simulink model "VIPL557LTStEnCtrl"  (R2024b)
settings: Solver=FixedStepDiscrete  StartTime=0.0  StopTime=10.0  RelTol=1e-3
undefined symbols (not defined in the file or in its folder): data, KeSMSw4SSecRwLtStLgrstUpwdDnwdOpenPos1_Val, SecRwLtStBkReclnEn_Clear, SecRwLtStBkReclnEn_Set, SecRwLtStFwdBkwdEn_Clear, SecRwLtStFwdBkwdEn_Set, SecRwLtStLgrstInwdOtwdEn_Clear, SecRwLtStLgrstInwdOtwdEn_Set, SecRwLtStLgrstUpwdDnwdEn_Clear, SecRwLtStLgrstUpwdDnwdEn_Set, ThdRwLtStBkReclnEn_Clear, ThdRwLtStBkReclnEn_Set, ThdRwLtStFwdBkwdEn_Clear, ThdRwLtStFwdBkwdEn_Set
libraries: simulink x1
settings Model: ModifiedHistory=2024.6.28 V3.0.0 座椅模式流程图V1.9  Creator=sn2xws  LastModifiedBy=sn55gm
settings SolverCC: AlgebraicLoopSolver=TrustRegion
settings DataIOCC: SaveFormat=StructureWithTime  ReturnWorkspaceOutputs=off
settings OptimizationCC: DefaultParameterBehavior=Inlined  EnhancedBackFolding=on  PassReuseOutputArgsAs=Individual arguments  ZeroExternalMemoryAtStartup=off  ZeroInternalMemoryAtStartup=off  OptimizeBlockOrder=speed  DifferentSizesBufferReuse=on  OptimizationCustomize=off  EfficientTunableParamExpr=on
settings DebuggingCC: ParameterTunabilityLossMsg=error  UnconnectedInputMsg=warning  UnconnectedOutputMsg=warning  UnconnectedLineMsg=warning  ArithmeticOperatorsInVariantConditions=warning
settings ModelReferenceCC: EnableRefExpFcnMdlSchedulingChecks=on
settings SFSimCC: MATLABDynamicMemAlloc=off  CustomCodeUndefinedFunction=UseInterfaceOnly
settings RTWCC: Description=AUTOSAR  SystemTargetFile=autosar.tlc  GenCodeOnly=on  TemplateMakefile=ert_default_tmf  GenerateReport=on  IncludeHyperlinkInReport=on  LaunchReport=on  DataTypeReplacement=CDataTypesFixedWidth  GenerateTraceInfo=on  GenerateTraceReport=on  GenerateTraceReportSl=on  GenerateTraceReportSf=on  GenerateTraceReportEml=on  GPUComputeCapability=3.5
settings CodeAppCC: ForceParamTrailComments=on  IgnoreCustomStorageClasses=off  OperatorAnnotations=on  SimulinkDataObjDesc=on  SFDataObjDesc=on  InsertBlockDesc=on
settings STFCustomTargetCC: TargetLangStandard=C99 (ISO)  MultiwordLength=256  ParMdlRefBuildCompliant=on  CompOptLevelCompliant=on  IncludeMdlTerminateFcn=off  CombineOutputUpdateFcns=on  SuppressErrorStatus=on  ERTCustomFileBanners=on  SupportNonFinite=off  SupportComplex=off  SupportContinuousTime=off  SupportNonInlinedSFcns=off  RemoveResetFunc=on  MATLABClassNameForMDSCustomization=Simulink.SoftwareTarget.ERTCustomization  AutosarCompliant=on  UseToolchainInfoCompliant=on  LookupTableObjectStructAxisOrder=2,1,3,4,...  LUTObjectStructOrderEvenSpacing=Size,Table,Breakpoints  SystemTargetFile=autosar.tlc
settings ERTTargetCC: TargetLangStandard=C99 (ISO)  ConcurrentExecutionCompliant=off  IncludeMdlTerminateFcn=off  SuppressErrorStatus=on  SupportNonFinite=off  SupportComplex=off  ModelStepFunctionPrototypeControlCompliant=off  CPPClassGenCompliant=off  AutosarCompliant=on  LookupTableObjectStructAxisOrder=2,1,3,4,...  LUTObjectStructOrderEvenSpacing=Size,Table,Breakpoints  ERTCustomFileTemplate=example_file_process.tlc  ERTFilePackagingFormat=Compact  BooleanTrueId=TRUE  BooleanFalseId=FALSE  DynamicArrayContainerType=coder::array

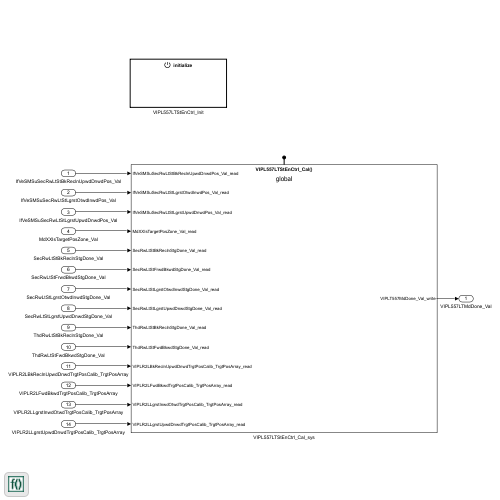
[thumbnail: Simulink's stored preview of the top-level diagram]
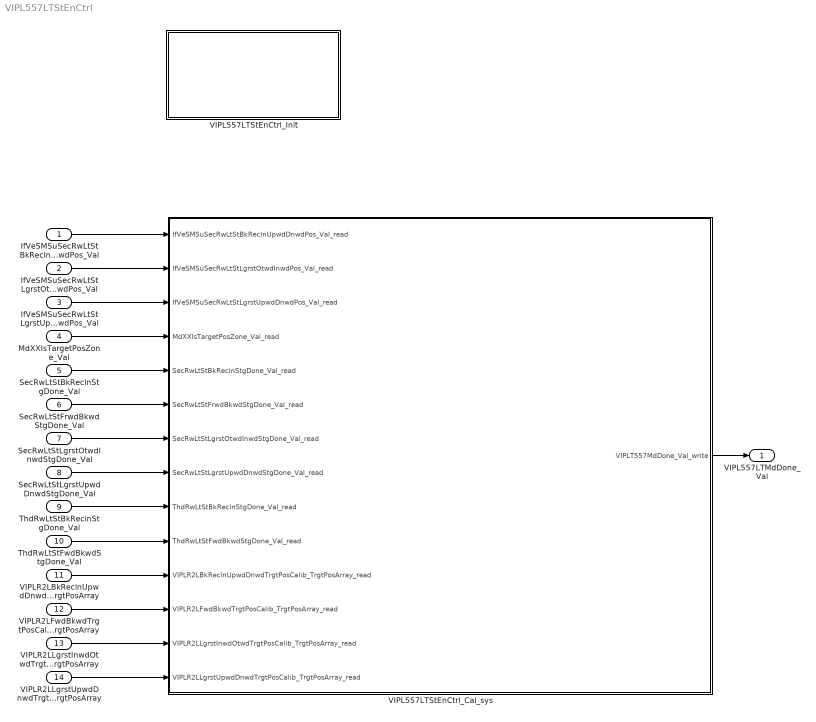
== system VIPL557LTStEnCtrl ==
  IfVeSMSuSecRwLtStBkReclnUpwdDnwdPos_Val : Inport  OutDataTypeStr=uint16  PortDimensions=1
  IfVeSMSuSecRwLtStLgrstOtwdInwdPos_Val : Inport  Port=2  OutDataTypeStr=uint16  PortDimensions=1
  IfVeSMSuSecRwLtStLgrstUpwdDnwdPos_Val : Inport  Port=3  OutDataTypeStr=uint16  PortDimensions=1
  MdXXIsTargetPosZone_Val : Inport  Port=4  OutDataTypeStr=uint32  PortDimensions=1
  SecRwLtStBkReclnStgDone_Val : Inport  Port=5  OutDataTypeStr=boolean  PortDimensions=1
  SecRwLtStFrwdBkwdStgDone_Val : Inport  Port=6  OutDataTypeStr=boolean  PortDimensions=1
  SecRwLtStLgrstOtwdInwdStgDone_Val : Inport  Port=7  OutDataTypeStr=boolean  PortDimensions=1
  SecRwLtStLgrstUpwdDnwdStgDone_Val : Inport  Port=8  OutDataTypeStr=boolean  PortDimensions=1
  ThdRwLtStBkReclnStgDone_Val : Inport  Port=9  OutDataTypeStr=boolean  PortDimensions=1
  ThdRwLtStFwdBkwdStgDone_Val : Inport  Port=10  OutDataTypeStr=boolean  PortDimensions=1
  VIPLR2LBkReclnUpwdDnwdTrgtPosCalib_TrgtPosArray : Inport  Description=|  Port=11  OutDataTypeStr=uint16  PortDimensions=3
      | 0:Pos
      | 1:Max
      | 2:Min
  VIPLR2LFwdBkwdTrgtPosCalib_TrgtPosArray : Inport  Description=|  Port=12  OutDataTypeStr=uint16  PortDimensions=3
      | 0:Pos
      | 1:Max
      | 2:Min
  VIPLR2LLgrstInwdOtwdTrgtPosCalib_TrgtPosArray : Inport  Description=|  Port=13  OutDataTypeStr=uint16  PortDimensions=3
      | 0:Pos
      | 1:Max
      | 2:Min
  VIPLR2LLgrstUpwdDnwdTrgtPosCalib_TrgtPosArray : Inport  Description=|  Port=14  OutDataTypeStr=uint16  PortDimensions=3
      | 0:Pos
      | 1:Max
      | 2:Min
  VIPL557LTStEnCtrl_Cal_sys : Subsystem
  VIPL557LTStEnCtrl_Init : Subsystem
  VIPL557LTMdDone_Val : Outport  OutDataTypeStr=uint8  PortDimensions=1  VectorParamsAs1DForOutWhenUnconnected=off
  wires:
  IfVeSMSuSecRwLtStBkReclnUpwdDnwdPos_Val/1 -> VIPL557LTStEnCtrl_Cal_sys/1(IfVeSMSuSecRwLtStBkReclnUpwdDnwdPos_Val_read)
  IfVeSMSuSecRwLtStLgrstOtwdInwdPos_Val/1 -> VIPL557LTStEnCtrl_Cal_sys/2(IfVeSMSuSecRwLtStLgrstOtwdInwdPos_Val_read)
  IfVeSMSuSecRwLtStLgrstUpwdDnwdPos_Val/1 -> VIPL557LTStEnCtrl_Cal_sys/3(IfVeSMSuSecRwLtStLgrstUpwdDnwdPos_Val_read)
  MdXXIsTargetPosZone_Val/1 -> VIPL557LTStEnCtrl_Cal_sys/4(MdXXIsTargetPosZone_Val_read)
  SecRwLtStBkReclnStgDone_Val/1 -> VIPL557LTStEnCtrl_Cal_sys/5(SecRwLtStBkReclnStgDone_Val_read)
  SecRwLtStFrwdBkwdStgDone_Val/1 -> VIPL557LTStEnCtrl_Cal_sys/6(SecRwLtStFrwdBkwdStgDone_Val_read)
  SecRwLtStLgrstOtwdInwdStgDone_Val/1 -> VIPL557LTStEnCtrl_Cal_sys/7(SecRwLtStLgrstOtwdInwdStgDone_Val_read)
  SecRwLtStLgrstUpwdDnwdStgDone_Val/1 -> VIPL557LTStEnCtrl_Cal_sys/8(SecRwLtStLgrstUpwdDnwdStgDone_Val_read)
  ThdRwLtStBkReclnStgDone_Val/1 -> VIPL557LTStEnCtrl_Cal_sys/9(ThdRwLtStBkReclnStgDone_Val_read)
  ThdRwLtStFwdBkwdStgDone_Val/1 -> VIPL557LTStEnCtrl_Cal_sys/10(ThdRwLtStFwdBkwdStgDone_Val_read)
  VIPLR2LBkReclnUpwdDnwdTrgtPosCalib_TrgtPosArray/1 -> VIPL557LTStEnCtrl_Cal_sys/11(VIPLR2LBkReclnUpwdDnwdTrgtPosCalib_TrgtPosArray_read)
  VIPLR2LFwdBkwdTrgtPosCalib_TrgtPosArray/1 -> VIPL557LTStEnCtrl_Cal_sys/12(VIPLR2LFwdBkwdTrgtPosCalib_TrgtPosArray_read)
  VIPLR2LLgrstInwdOtwdTrgtPosCalib_TrgtPosArray/1 -> VIPL557LTStEnCtrl_Cal_sys/13(VIPLR2LLgrstInwdOtwdTrgtPosCalib_TrgtPosArray_read)
  VIPLR2LLgrstUpwdDnwdTrgtPosCalib_TrgtPosArray/1 -> VIPL557LTStEnCtrl_Cal_sys/14(VIPLR2LLgrstUpwdDnwdTrgtPosCalib_TrgtPosArray_read)
  VIPL557LTStEnCtrl_Cal_sys/1(VIPLT557MdDone_Val_write) -> VIPL557LTMdDone_Val/1

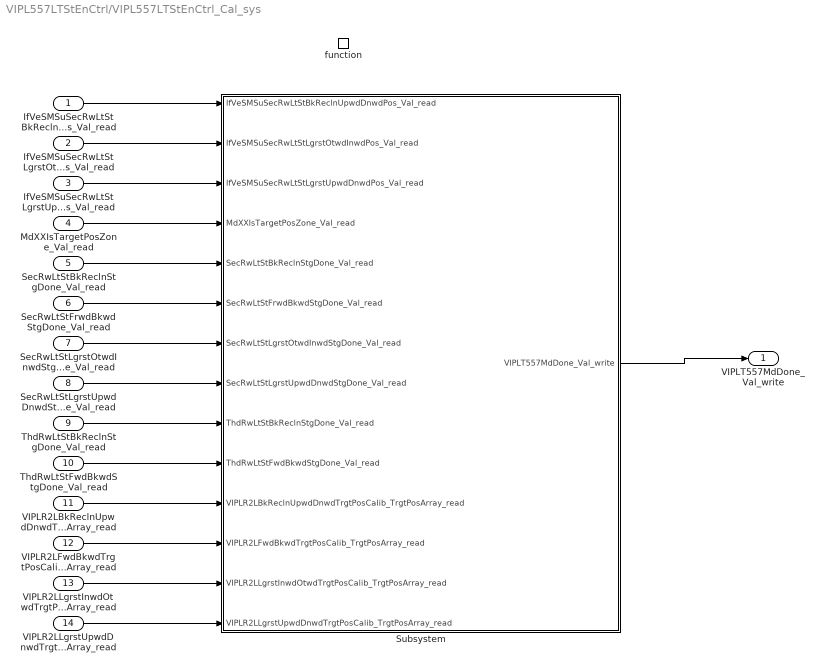
== system VIPL557LTStEnCtrl/VIPL557LTStEnCtrl_Cal_sys ==
  IfVeSMSuSecRwLtStBkReclnUpwdDnwdPos_Val_read : Inport
  IfVeSMSuSecRwLtStLgrstOtwdInwdPos_Val_read : Inport  Port=2
  IfVeSMSuSecRwLtStLgrstUpwdDnwdPos_Val_read : Inport  Port=3
  MdXXIsTargetPosZone_Val_read : Inport  Port=4
  SecRwLtStBkReclnStgDone_Val_read : Inport  Port=5
  SecRwLtStFrwdBkwdStgDone_Val_read : Inport  Port=6
  SecRwLtStLgrstOtwdInwdStgDone_Val_read : Inport  Port=7
  SecRwLtStLgrstUpwdDnwdStgDone_Val_read : Inport  Port=8
  ThdRwLtStBkReclnStgDone_Val_read : Inport  Port=9
  ThdRwLtStFwdBkwdStgDone_Val_read : Inport  Port=10
  VIPLR2LBkReclnUpwdDnwdTrgtPosCalib_TrgtPosArray_read : Inport  Port=11
  VIPLR2LFwdBkwdTrgtPosCalib_TrgtPosArray_read : Inport  Port=12
  VIPLR2LLgrstInwdOtwdTrgtPosCalib_TrgtPosArray_read : Inport  Port=13
  VIPLR2LLgrstUpwdDnwdTrgtPosCalib_TrgtPosArray_read : Inport  Port=14
  function : TriggerPort  TriggerType=function-call  IsSimulinkFunction=on  FunctionName=VIPL557LTStEnCtrl_Cal  VariantControl=(inherit)
  Subsystem : Subsystem
  VIPLT557MdDone_Val_write : Outport  VectorParamsAs1DForOutWhenUnconnected=off
      settings: EnsureOutportIsVirtual=on
  wires:
  IfVeSMSuSecRwLtStBkReclnUpwdDnwdPos_Val_read/1 -> Subsystem/1(IfVeSMSuSecRwLtStBkReclnUpwdDnwdPos_Val_read)
  IfVeSMSuSecRwLtStLgrstOtwdInwdPos_Val_read/1 -> Subsystem/2(IfVeSMSuSecRwLtStLgrstOtwdInwdPos_Val_read)
  IfVeSMSuSecRwLtStLgrstUpwdDnwdPos_Val_read/1 -> Subsystem/3(IfVeSMSuSecRwLtStLgrstUpwdDnwdPos_Val_read)
  MdXXIsTargetPosZone_Val_read/1 -> Subsystem/4(MdXXIsTargetPosZone_Val_read)
  SecRwLtStBkReclnStgDone_Val_read/1 -> Subsystem/5(SecRwLtStBkReclnStgDone_Val_read)
  SecRwLtStFrwdBkwdStgDone_Val_read/1 -> Subsystem/6(SecRwLtStFrwdBkwdStgDone_Val_read)
  SecRwLtStLgrstOtwdInwdStgDone_Val_read/1 -> Subsystem/7(SecRwLtStLgrstOtwdInwdStgDone_Val_read)
  SecRwLtStLgrstUpwdDnwdStgDone_Val_read/1 -> Subsystem/8(SecRwLtStLgrstUpwdDnwdStgDone_Val_read)
  ThdRwLtStBkReclnStgDone_Val_read/1 -> Subsystem/9(ThdRwLtStBkReclnStgDone_Val_read)
  ThdRwLtStFwdBkwdStgDone_Val_read/1 -> Subsystem/10(ThdRwLtStFwdBkwdStgDone_Val_read)
  VIPLR2LBkReclnUpwdDnwdTrgtPosCalib_TrgtPosArray_read/1 -> Subsystem/11(VIPLR2LBkReclnUpwdDnwdTrgtPosCalib_TrgtPosArray_read)
  VIPLR2LFwdBkwdTrgtPosCalib_TrgtPosArray_read/1 -> Subsystem/12(VIPLR2LFwdBkwdTrgtPosCalib_TrgtPosArray_read)
  VIPLR2LLgrstInwdOtwdTrgtPosCalib_TrgtPosArray_read/1 -> Subsystem/13(VIPLR2LLgrstInwdOtwdTrgtPosCalib_TrgtPosArray_read)
  VIPLR2LLgrstUpwdDnwdTrgtPosCalib_TrgtPosArray_read/1 -> Subsystem/14(VIPLR2LLgrstUpwdDnwdTrgtPosCalib_TrgtPosArray_read)
  Subsystem/1(VIPLT557MdDone_Val_write) -> VIPLT557MdDone_Val_write/1

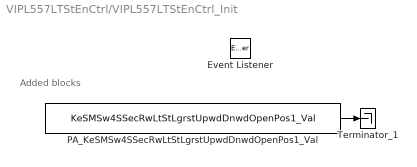
== system VIPL557LTStEnCtrl/VIPL557LTStEnCtrl_Init ==
  note: Added blocks
  Event Listener : EventListener  EventName=reset
  PA_KeSMSw4SSecRwLtStLgrstUpwdDnwdOpenPos1_Val : Constant  Value=KeSMSw4SSecRwLtStLgrstUpwdDnwdOpenPos1_Val
  Terminator_1 : Terminator
  wires:
  PA_KeSMSw4SSecRwLtStLgrstUpwdDnwdOpenPos1_Val/1 -> Terminator_1/1

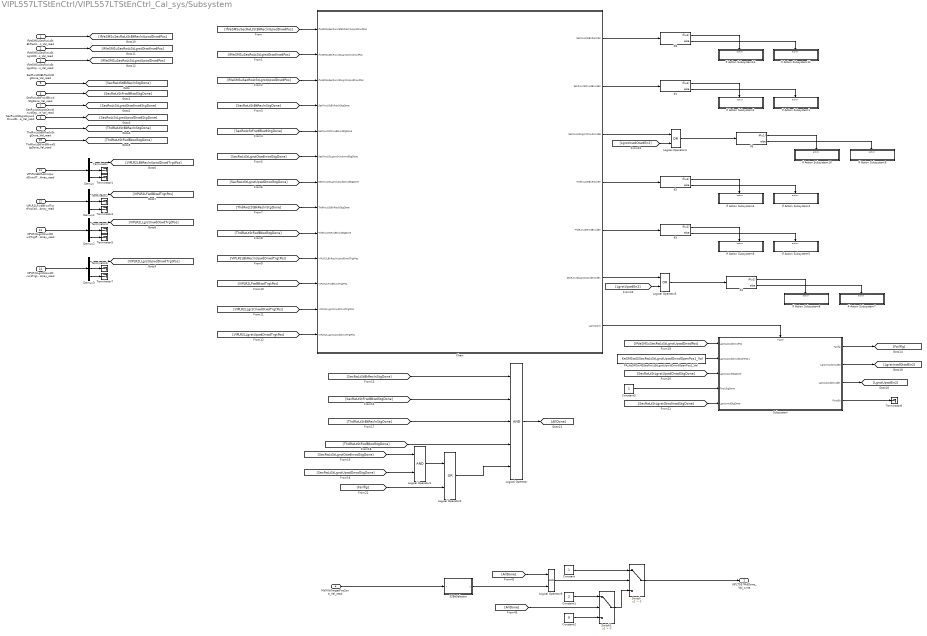
== system VIPL557LTStEnCtrl/VIPL557LTStEnCtrl_Cal_sys/Subsystem ==
  IfVeSMSuSecRwLtStBkReclnUpwdDnwdPos_Val_read : Inport
  IfVeSMSuSecRwLtStLgrstOtwdInwdPos_Val_read : Inport  Port=2
  IfVeSMSuSecRwLtStLgrstUpwdDnwdPos_Val_read : Inport  Port=3
  MdXXIsTargetPosZone_Val_read : Inport  Port=4
  SecRwLtStBkReclnStgDone_Val_read : Inport  Port=5
  SecRwLtStFrwdBkwdStgDone_Val_read : Inport  Port=6
  SecRwLtStLgrstOtwdInwdStgDone_Val_read : Inport  Port=7
  SecRwLtStLgrstUpwdDnwdStgDone_Val_read : Inport  Port=8
  ThdRwLtStBkReclnStgDone_Val_read : Inport  Port=9
  ThdRwLtStFwdBkwdStgDone_Val_read : Inport  Port=10
  VIPLR2LBkReclnUpwdDnwdTrgtPosCalib_TrgtPosArray_read : Inport  Port=11
  VIPLR2LFwdBkwdTrgtPosCalib_TrgtPosArray_read : Inport  Port=12
  VIPLR2LLgrstInwdOtwdTrgtPosCalib_TrgtPosArray_read : Inport  Port=13
  VIPLR2LLgrstUpwdDnwdTrgtPosCalib_TrgtPosArray_read : Inport  Port=14
  32BitSelector : Subsystem  mask(32 Bit Selector){BitNum=9}
      mask prompts: BitNum "Select Bit Number"
      mask help: Allows selection of a particular bit (0-31) out of a packed word up to 32 bits long. Output will be true if the bit number selected via the mask parameter is equal to one.
      mask TypeOptions BitNum: 0 | 1 | 2 | 3 | 4 | 5 | 6 | 7 | 8 | 9 | 10 | 11 | 12 | 13 | 14 | 15 | 16 | 17 | 18 | 19 | 20 | 21 | 22 | 23 | 24 | 25 | 26 | 27 | 28 | 29 | 30 | 31
      mask Display:
      | text(0.5, 0.8,'BIT','horizontalAlignment','center')
      | text(0.5, 0.5,'SELECTOR','horizontalAlignment','center')
      | text(0.5, 0.2,['-- Bit ',char(get_param(gcb,'BitNum')),' --'],'horizontalAlignment','center')
  Chart : Stateflow chart  TreatAsAtomicUnit=on
  Constant : Constant  OutDataTypeStr=uint8
  Constant1 : Constant  Value=2  OutDataTypeStr=uint8
  Constant2 : Constant  Value=0  OutDataTypeStr=uint8
  Constant3 : Constant  OutDataTypeStr=boolean
  Demux{,1..3} (4 alike) : Demux  Outputs=3
  If Action Subsystem1 : Subsystem  TreatAsAtomicUnit=on
  If Action Subsystem10 : Subsystem  TreatAsAtomicUnit=on
  If Action Subsystem11 : Subsystem  TreatAsAtomicUnit=on
  If Action Subsystem14 : Subsystem  TreatAsAtomicUnit=on
  If Action Subsystem2 : Subsystem  TreatAsAtomicUnit=on
  If Action Subsystem3 : Subsystem  TreatAsAtomicUnit=on
  If Action Subsystem4 : Subsystem  TreatAsAtomicUnit=on
  If Action Subsystem5 : Subsystem  TreatAsAtomicUnit=on
  If Action Subsystem6 : Subsystem  TreatAsAtomicUnit=on
  If Action Subsystem7 : Subsystem  TreatAsAtomicUnit=on
  If Action Subsystem8 : Subsystem  TreatAsAtomicUnit=on
  If Action Subsystem9 : Subsystem  TreatAsAtomicUnit=on
  If{1..5,8} (6 alike) : If  IfExpression=u1
  Logical Operator : Logic  Inputs=5  AllPortsSameDT=off  OutDataTypeStr=boolean
  Logical Operator1 : Logic  AllPortsSameDT=off  OutDataTypeStr=boolean
  Logical Operator2 : Logic  Operator=OR  AllPortsSameDT=off  OutDataTypeStr=boolean
  Logical Operator3 : Logic  Operator=OR  AllPortsSameDT=off  OutDataTypeStr=boolean
  Logical Operator4 : Logic  Operator=OR  AllPortsSameDT=off  OutDataTypeStr=boolean
  Logical Operator9 : Logic  AllPortsSameDT=off  OutDataTypeStr=boolean
  PA_KeSMSw4SSecRwLtStLgrstUpwdDnwdOpenPos1_Val : Constant  Value=KeSMSw4SSecRwLtStLgrstUpwdDnwdOpenPos1_Val
  Subsystem : Subsystem
  Switch : Switch  Criteria=u2 > Threshold  SaturateOnIntegerOverflow=off  InputSameDT=off
  Switch1 : Switch  Criteria=u2 > Threshold  SaturateOnIntegerOverflow=off  InputSameDT=off
  Terminator{,1..8} (9 alike) : Terminator
  VIPLT557MdDone_Val_write : Outport  VectorParamsAs1DForOutWhenUnconnected=off
      settings: EnsureOutportIsVirtual=on
  wires:
  Switch/1 -> VIPLT557MdDone_Val_write/1
  SecRwLtStBkReclnStgDone_Val_read/1 -> [SecRwLtStBkReclnStgDone]
  SecRwLtStFrwdBkwdStgDone_Val_read/1 -> [SecRwLtStFrwdBkwdStgDone]
  SecRwLtStLgrstOtwdInwdStgDone_Val_read/1 -> [SecRwLtStLgrstOtwdInwdStgDone]
  SecRwLtStLgrstUpwdDnwdStgDone_Val_read/1 -> [SecRwLtStLgrstUpwdDnwdStgDone]
  ThdRwLtStBkReclnStgDone_Val_read/1 -> [ThdRwLtStBkReclnStgDone]
  ThdRwLtStFwdBkwdStgDone_Val_read/1 -> [ThdRwLtStFwdBkwdStgDone]
  VIPLR2LBkReclnUpwdDnwdTrgtPosCalib_TrgtPosArray_read/1 -> Demux/1
  Demux/1 -> [VIPLR2LBkReclnUpwdDnwdTrgtPos]
  Demux/2 -> Terminator/1
  Demux/3 -> Terminator1/1
  Demux1/3 -> Terminator3/1
  Demux1/2 -> Terminator2/1
  Demux1/1 -> [VIPLR2LFwdBkwdTrgtPos]
  VIPLR2LFwdBkwdTrgtPosCalib_TrgtPosArray_read/1 -> Demux1/1
  VIPLR2LLgrstInwdOtwdTrgtPosCalib_TrgtPosArray_read/1 -> Demux2/1
  Demux2/1 -> [VIPLR2LLgrstInwdOtwdTrgtPos]
  Demux2/2 -> Terminator4/1
  Demux2/3 -> Terminator5/1
  Demux3/3 -> Terminator7/1
  Demux3/2 -> Terminator6/1
  Demux3/1 -> [VIPLR2LLgrstUpwdDnwdTrgtPos]
  VIPLR2LLgrstUpwdDnwdTrgtPosCalib_TrgtPosArray_read/1 -> Demux3/1
  IfVeSMSuSecRwLtStBkReclnUpwdDnwdPos_Val_read/1 -> [IfVeSMSuSecRwLtStBkReclnUpwdDnwdPos]
  IfVeSMSuSecRwLtStLgrstOtwdInwdPos_Val_read/1 -> [IfVeSMSuSecRwLtStLgrstOtwdInwdPos]
  IfVeSMSuSecRwLtStLgrstUpwdDnwdPos_Val_read/1 -> [IfVeSMSuSecRwLtStLgrstUpwdDnwdPos]
  [IfVeSMSuSecRwLtStBkReclnUpwdDnwdPos] -> Chart/1(IfVeSMSuSecRwLtStBkReclnUpwdDnwdPos)
  [IfVeSMSuSecRwLtStLgrstOtwdInwdPos] -> Chart/2(IfVeSMSuSecRwLtStLgrstOtwdInwdPos)
  [IfVeSMSuSecRwLtStLgrstUpwdDnwdPos] -> Chart/3(IfVeSMSuSecRwLtStLgrstUpwdDnwdPos)
  [SecRwLtStBkReclnStgDone] -> Chart/4(SecRwLtStBkReclnStgDone)
  [SecRwLtStFrwdBkwdStgDone] -> Chart/5(SecRwLtStFrwdBkwdStgDone)
  [SecRwLtStLgrstOtwdInwdStgDone] -> Chart/6(SecRwLtStLgrstOtwdInwdStgDone)
  [SecRwLtStLgrstUpwdDnwdStgDone] -> Chart/7(SecRwLtStLgrstUpwdDnwdStgDone)
  [ThdRwLtStBkReclnStgDone] -> Chart/8(ThdRwLtStBkReclnStgDone)
  [ThdRwLtStFwdBkwdStgDone] -> Chart/9(ThdRwLtStFwdBkwdStgDone)
  [VIPLR2LBkReclnUpwdDnwdTrgtPos] -> Chart/10(VIPLR2LBkReclnUpwdDnwdTrgtPos)
  [VIPLR2LFwdBkwdTrgtPos] -> Chart/11(VIPLR2LFwdBkwdTrgtPos)
  [VIPLR2LLgrstInwdOtwdTrgtPos] -> Chart/12(VIPLR2LLgrstInwdOtwdTrgtPos)
  [VIPLR2LLgrstUpwdDnwdTrgtPos] -> Chart/13(VIPLR2LLgrstUpwdDnwdTrgtPos)
  [SecRwLtStBkReclnStgDone] -> Logical Operator/1
  [SecRwLtStFrwdBkwdStgDone] -> Logical Operator/2
  [AllDone] -> Switch1/2
  MdXXIsTargetPosZone_Val_read/1 -> 32BitSelector/1(x)
  32BitSelector/1(y) -> Logical Operator9/2
  Constant/1 -> Switch/1
  Logical Operator9/1 -> Switch/2
  Switch1/1 -> Switch/3
  Constant1/1 -> Switch1/1
  [AllDone] -> Logical Operator9/1
  Constant2/1 -> Switch1/3
  Logical Operator/1 -> [AllDone]
  Chart/7(LgrstOpn()) -> Subsystem/Trigger
  [IfVeSMSuSecRwLtStLgrstUpwdDnwdPos] -> Subsystem/1(LgrstUpwdDnwdPos)
  [SecRwLtStLgrstUpwdDnwdStgDone] -> Subsystem/3(LgrstUpwdStgDone)
  Constant3/1 -> Subsystem/4(FtrstStgDone)
  [SecRwLtStLgrstOtwdInwdStgDone] -> Subsystem/5(LgrstInwdStgDone)
  Subsystem/1(Failflg) -> [Failflg]
  Subsystem/4(FtrstEn) -> Terminator8/1
  [SecRwLtStLgrstOtwdInwdStgDone] -> Logical Operator1/1
  [SecRwLtStLgrstUpwdDnwdStgDone] -> Logical Operator1/2
  [Failflg] -> Logical Operator2/2
  Logical Operator1/1 -> Logical Operator2/1
  [ThdRwLtStBkReclnStgDone] -> Logical Operator/3
  [ThdRwLtStFwdBkwdStgDone] -> Logical Operator/4
  Logical Operator2/1 -> Logical Operator/5
  If8/2 -> If Action Subsystem11/Action
  If8/1 -> If Action Subsystem14/Action
  Chart/1(SecRwLtStBkReclnEn) -> If8/1
  Chart/2(SecRwLtStFrwdBkwdEn) -> If1/1
  If1/1 -> If Action Subsystem2/Action
  If1/2 -> If Action Subsystem1/Action
  If2/2 -> If Action Subsystem3/Action
  If2/1 -> If Action Subsystem4/Action
  Chart/4(ThdRwLtStBkReclnEn) -> If2/1
  Chart/5(ThdRwLtStFwdBkwdEn) -> If3/1
  If3/1 -> If Action Subsystem6/Action
  If3/2 -> If Action Subsystem5/Action
  Chart/6(SecRwLtStLgrstUpwdDnwdEn) -> Logical Operator3/1
  Subsystem/3(LgrstUpwdDnwdEn) -> [LgrstUpwdEn2]
  Chart/3(SecRwLtStLgrstOtwdInwdEn) -> Logical Operator4/1
  Subsystem/2(LgrstInwdOtwdEn) -> [LgrstInwdOtwdEn2]
  [LgrstUpwdEn2] -> Logical Operator3/2
  If4/2 -> If Action Subsystem7/Action
  If4/1 -> If Action Subsystem8/Action
  Logical Operator3/1 -> If4/1
  [LgrstInwdOtwdEn2] -> Logical Operator4/2
  Logical Operator4/1 -> If5/1
  If5/1 -> If Action Subsystem10/Action
  If5/2 -> If Action Subsystem9/Action
  PA_KeSMSw4SSecRwLtStLgrstUpwdDnwdOpenPos1_Val/1 -> Subsystem/2(LgrstUpwdDnwdOpenPos1)

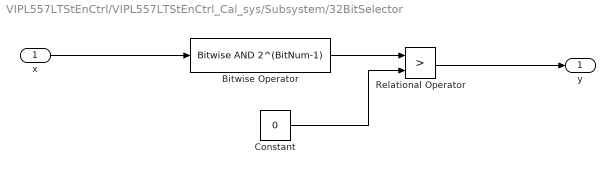
== system VIPL557LTStEnCtrl/VIPL557LTStEnCtrl_Cal_sys/Subsystem/32BitSelector ==
  x : Inport
  Bitwise Operator : simulink/Logic and Bit Operations/Bitwise Operator  logicop=AND  UseBitMask=on  BitMask=2^(BitNum-1)  BitMaskRealWorld=Stored Integer
  Constant : Constant  Value=0  OutDataTypeStr=uint32
  Relational Operator : RelationalOperator  Operator=>  OutDataTypeStr=boolean  RndMeth=Simplest  InputSameDT=off
  y : Outport  VectorParamsAs1DForOutWhenUnconnected=off
  wires:
  Relational Operator/1 -> y/1
  Constant/1 -> Relational Operator/2
  x/1 -> Bitwise Operator/1
  Bitwise Operator/1 -> Relational Operator/1

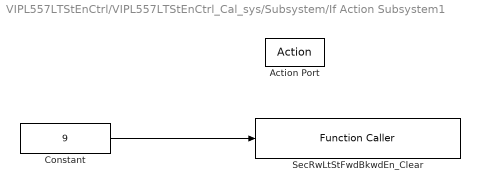
== system VIPL557LTStEnCtrl/VIPL557LTStEnCtrl_Cal_sys/Subsystem/If Action Subsystem1 ==
  Action Port : ActionPort  ActionPortLabel=else { }
  Constant : Constant  Value=9  OutDataTypeStr=uint8
  SecRwLtStFwdBkwdEn_Clear : FunctionCaller  FunctionPrototype=SecRwLtStFwdBkwdEn_Clear(data)  InputArgumentSpecifications=uint8(1)  OutputArgumentSpecifications=<Enter example>
  wires:
  Constant/1 -> SecRwLtStFwdBkwdEn_Clear/1

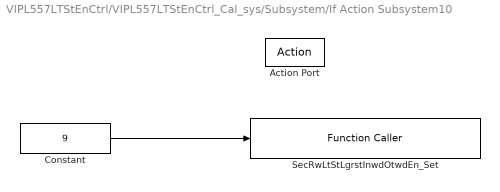
== system VIPL557LTStEnCtrl/VIPL557LTStEnCtrl_Cal_sys/Subsystem/If Action Subsystem10 ==
  Action Port : ActionPort  ActionPortLabel=if { }
  Constant : Constant  Value=9  OutDataTypeStr=uint8
  SecRwLtStLgrstInwdOtwdEn_Set : FunctionCaller  FunctionPrototype=SecRwLtStLgrstInwdOtwdEn_Set(data)  InputArgumentSpecifications=uint8(1)  OutputArgumentSpecifications=<Enter example>
  wires:
  Constant/1 -> SecRwLtStLgrstInwdOtwdEn_Set/1

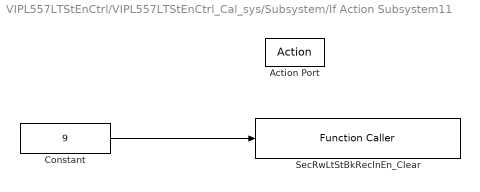
== system VIPL557LTStEnCtrl/VIPL557LTStEnCtrl_Cal_sys/Subsystem/If Action Subsystem11 ==
  Action Port : ActionPort  ActionPortLabel=else { }
  Constant : Constant  Value=9  OutDataTypeStr=uint8
  SecRwLtStBkReclnEn_Clear : FunctionCaller  FunctionPrototype=SecRwLtStBkReclnEn_Clear(data)  InputArgumentSpecifications=uint8(1)  OutputArgumentSpecifications=<Enter example>
  wires:
  Constant/1 -> SecRwLtStBkReclnEn_Clear/1

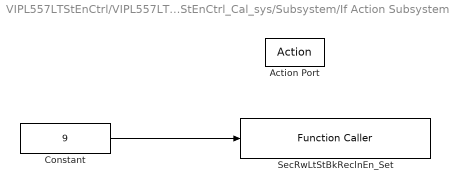
== system VIPL557LTStEnCtrl/VIPL557LTStEnCtrl_Cal_sys/Subsystem/If Action Subsystem14 ==
  Action Port : ActionPort  ActionPortLabel=if { }
  Constant : Constant  Value=9  OutDataTypeStr=uint8
  SecRwLtStBkReclnEn_Set : FunctionCaller  FunctionPrototype=SecRwLtStBkReclnEn_Set(data)  InputArgumentSpecifications=uint8(1)  OutputArgumentSpecifications=<Enter example>
  wires:
  Constant/1 -> SecRwLtStBkReclnEn_Set/1

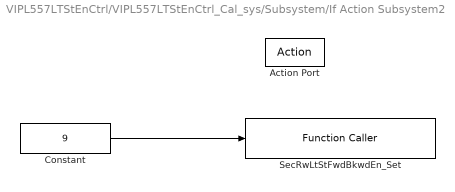
== system VIPL557LTStEnCtrl/VIPL557LTStEnCtrl_Cal_sys/Subsystem/If Action Subsystem2 ==
  Action Port : ActionPort  ActionPortLabel=if { }
  Constant : Constant  Value=9  OutDataTypeStr=uint8
  SecRwLtStFwdBkwdEn_Set : FunctionCaller  FunctionPrototype=SecRwLtStFwdBkwdEn_Set(data)  InputArgumentSpecifications=uint8(1)  OutputArgumentSpecifications=<Enter example>
  wires:
  Constant/1 -> SecRwLtStFwdBkwdEn_Set/1

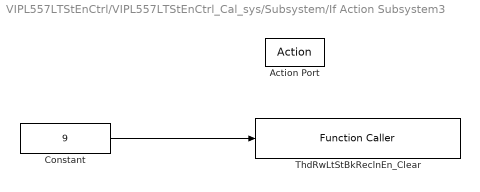
== system VIPL557LTStEnCtrl/VIPL557LTStEnCtrl_Cal_sys/Subsystem/If Action Subsystem3 ==
  Action Port : ActionPort  ActionPortLabel=else { }
  Constant : Constant  Value=9  OutDataTypeStr=uint8
  ThdRwLtStBkReclnEn_Clear : FunctionCaller  FunctionPrototype=ThdRwLtStBkReclnEn_Clear(data)  InputArgumentSpecifications=uint8(1)  OutputArgumentSpecifications=<Enter example>
  wires:
  Constant/1 -> ThdRwLtStBkReclnEn_Clear/1

== system VIPL557LTStEnCtrl/VIPL557LTStEnCtrl_Cal_sys/Subsystem/If Action Subsystem4 ==
  Action Port : ActionPort  ActionPortLabel=if { }
  Constant : Constant  Value=9  OutDataTypeStr=uint8
  ThdRwLtStBkReclnEn_Set : FunctionCaller  FunctionPrototype=ThdRwLtStBkReclnEn_Set(data)  InputArgumentSpecifications=uint8(1)  OutputArgumentSpecifications=<Enter example>
  wires:
  Constant/1 -> ThdRwLtStBkReclnEn_Set/1

== system VIPL557LTStEnCtrl/VIPL557LTStEnCtrl_Cal_sys/Subsystem/If Action Subsystem5 ==
  Action Port : ActionPort  ActionPortLabel=else { }
  Constant : Constant  Value=9  OutDataTypeStr=uint8
  ThdRwLtStFwdBkwdEn_Clear : FunctionCaller  FunctionPrototype=ThdRwLtStFwdBkwdEn_Clear(data)  InputArgumentSpecifications=uint8(1)  OutputArgumentSpecifications=<Enter example>
  wires:
  Constant/1 -> ThdRwLtStFwdBkwdEn_Clear/1

== system VIPL557LTStEnCtrl/VIPL557LTStEnCtrl_Cal_sys/Subsystem/If Action Subsystem6 ==
  Action Port : ActionPort  ActionPortLabel=if { }
  Constant : Constant  Value=9  OutDataTypeStr=uint8
  ThdRwLtStFwdBkwdEn_Set : FunctionCaller  FunctionPrototype=ThdRwLtStFwdBkwdEn_Set(data)  InputArgumentSpecifications=uint8(1)  OutputArgumentSpecifications=<Enter example>
  wires:
  Constant/1 -> ThdRwLtStFwdBkwdEn_Set/1

== system VIPL557LTStEnCtrl/VIPL557LTStEnCtrl_Cal_sys/Subsystem/If Action Subsystem7 ==
  Action Port : ActionPort  ActionPortLabel=else { }
  Constant : Constant  Value=9  OutDataTypeStr=uint8
  SecRwLtStLgrstUpwdDnwdEn_Clear : FunctionCaller  FunctionPrototype=SecRwLtStLgrstUpwdDnwdEn_Clear(data)  InputArgumentSpecifications=uint8(1)  OutputArgumentSpecifications=<Enter example>
  wires:
  Constant/1 -> SecRwLtStLgrstUpwdDnwdEn_Clear/1

== system VIPL557LTStEnCtrl/VIPL557LTStEnCtrl_Cal_sys/Subsystem/If Action Subsystem8 ==
  Action Port : ActionPort  ActionPortLabel=if { }
  Constant : Constant  Value=9  OutDataTypeStr=uint8
  SecRwLtStLgrstUpwdDnwdEn_Set : FunctionCaller  FunctionPrototype=SecRwLtStLgrstUpwdDnwdEn_Set(data)  InputArgumentSpecifications=uint8(1)  OutputArgumentSpecifications=<Enter example>
  wires:
  Constant/1 -> SecRwLtStLgrstUpwdDnwdEn_Set/1

== system VIPL557LTStEnCtrl/VIPL557LTStEnCtrl_Cal_sys/Subsystem/If Action Subsystem9 ==
  Action Port : ActionPort  ActionPortLabel=else { }
  Constant : Constant  Value=9  OutDataTypeStr=uint8
  SecRwLtStLgrstInwdOtwdEn_Clear : FunctionCaller  FunctionPrototype=SecRwLtStLgrstInwdOtwdEn_Clear(data)  InputArgumentSpecifications=uint8(1)  OutputArgumentSpecifications=<Enter example>
  wires:
  Constant/1 -> SecRwLtStLgrstInwdOtwdEn_Clear/1

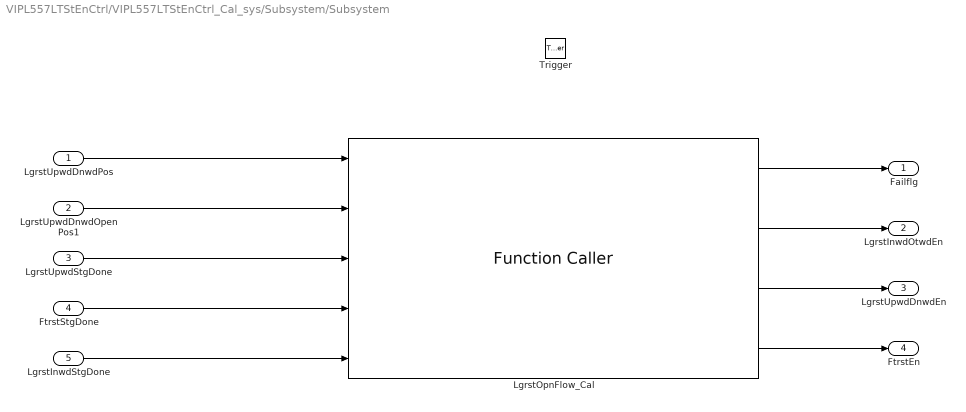
== system VIPL557LTStEnCtrl/VIPL557LTStEnCtrl_Cal_sys/Subsystem/Subsystem ==
  LgrstUpwdDnwdPos : Inport
  LgrstUpwdDnwdOpenPos1 : Inport  Port=2
  LgrstUpwdStgDone : Inport  Port=3
  FtrstStgDone : Inport  Port=4
  LgrstInwdStgDone : Inport  Port=5
  Trigger : TriggerPort  TriggerType=function-call  VariantControl=Variant  PortDimensions=1
  LgrstOpnFlow_Cal : FunctionCaller  FunctionPrototype=[Failflg,LgrstInwdOtwdEn,LgrstUpwdDnwdEn,FtrstEn] = LgrstOpnFlow_Cal(LgrstUpwdDnwdPos,LgrstUpwdDnwdOpenPos1,LgrstUpwdStgDone,FtrstStgDone,LgrstInwdStgDone)  InputArgumentSpecifications=uint16(1), uint16(1), boolean(true), boolean(true), boolean(true)  OutputArgumentSpecifications=boolean(true), boolean(true), boolean(true), boolean(true)
  Failflg : Outport  VectorParamsAs1DForOutWhenUnconnected=off
  LgrstInwdOtwdEn : Outport  Port=2  VectorParamsAs1DForOutWhenUnconnected=off
  LgrstUpwdDnwdEn : Outport  Port=3  VectorParamsAs1DForOutWhenUnconnected=off
  FtrstEn : Outport  Port=4  VectorParamsAs1DForOutWhenUnconnected=off
  wires:
  LgrstOpnFlow_Cal/2 -> LgrstInwdOtwdEn/1
  LgrstUpwdDnwdPos/1 -> LgrstOpnFlow_Cal/1
  LgrstOpnFlow_Cal/3 -> LgrstUpwdDnwdEn/1
  FtrstStgDone/1 -> LgrstOpnFlow_Cal/4
  LgrstUpwdStgDone/1 -> LgrstOpnFlow_Cal/3
  LgrstOpnFlow_Cal/4 -> FtrstEn/1
  LgrstInwdStgDone/1 -> LgrstOpnFlow_Cal/5
  LgrstUpwdDnwdOpenPos1/1 -> LgrstOpnFlow_Cal/2
  LgrstOpnFlow_Cal/1 -> Failflg/1

== stateflow chart VIPL557LTStEnCtrl/VIPL557LTStEnCtrl_Cal_sys/Subsystem/Chart ==
  (default) -> (junction 1) : {
      | ThdRwLtStBkReclnEn = 0;
      | SecRwLtStBkReclnEn = 0;
      | SecRwLtStFrwdBkwdEn = 0;
      | SecRwLtStLgrstOtwdInwdEn = 0;
      | SecRwLtStLgrstUpwdDnwdEn = 0;
      | ThdRwLtStFwdBkwdEn = 0;
      | }
  (junction 1) -> (junction 22) [order 1] : [!ThdRwLtStBkReclnStgDone]
  (junction 1) -> (junction 103) [order 2]
  (junction 22) -> (junction 24) : {ThdRwLtStBkReclnEn = 1;}
  (junction 103) -> (junction 98) [order 1] : [!ThdRwLtStFwdBkwdStgDone]
  (junction 98) -> (junction 97) : {ThdRwLtStFwdBkwdEn = 1;}
  (junction 103) -> (junction 26) [order 2]
  (junction 24) -> (junction 26)
  (junction 26) -> (junction 38)
  (junction 38) -> (junction 40) [order 1] : [IfVeSMSuSecRwLtStBkReclnUpwdDnwdPos>VIPLR2LBkReclnUpwdDnwdTrgtPos&&!SecRwLtStBkReclnStgDone]
  (junction 38) -> (junction 44) [order 2]
  (junction 40) -> (junction 42) : {SecRwLtStBkReclnEn = 1;}
  (junction 42) -> (junction 44)
  (junction 44) -> (junction 47)
  (junction 47) -> (junction 49) [order 1] : [IfVeSMSuSecRwLtStLgrstOtwdInwdPos >VIPLR2LLgrstInwdOtwdTrgtPos &&!SecRwLtStLgrstOtwdInwdStgDone]
  (junction 47) -> (junction 53) [order 2]
  (junction 49) -> (junction 51) : {SecRwLtStLgrstOtwdInwdEn = 1;}
  (junction 51) -> (junction 53)
  (junction 53) -> (junction 56)
  (junction 56) -> (junction 58) [order 1] : [IfVeSMSuSecRwLtStLgrstUpwdDnwdPos >VIPLR2LLgrstUpwdDnwdTrgtPos && !SecRwLtStLgrstUpwdDnwdStgDone]
  (junction 56) -> (junction 62) [order 2]
  (junction 58) -> (junction 60) : {SecRwLtStLgrstUpwdDnwdEn = 1;}
  (junction 60) -> (junction 62)
  (junction 62) -> (junction 65)
  (junction 65) -> (junction 67) [order 1] : [(IfVeSMSuSecRwLtStBkReclnUpwdDnwdPos<=VIPLR2LBkReclnUpwdDnwdTrgtPos||SecRwLtStBkReclnStgDone)&&...
      | (IfVeSMSuSecRwLtStLgrstOtwdInwdPos <=VIPLR2LLgrstInwdOtwdTrgtPos ||SecRwLtStLgrstOtwdInwdStgDone) &&...
      | (IfVeSMSuSecRwLtStLgrstUpwdDnwdPos <=VIPLR2LLgrstUpwdDnwdTrgtPos ||SecRwLtStLgrstUpwdDnwdStgDone)]
  (junction 67) -> (junction 69) [order 1] : [SecRwLtStFrwdBkwdStgDone]
  (junction 69) -> (junction 76) [order 1] : [SecRwLtStBkReclnStgDone]
  (junction 65) -> (junction 87) [order 2]
  (junction 67) -> (junction 73) [order 2] : {SecRwLtStFrwdBkwdEn =1;}
  (junction 69) -> (junction 71) [order 2] : {SecRwLtStBkReclnEn = 1;}
  (junction 76) -> (junction 78)
  (junction 78) -> (junction 71)
  (junction 71) -> (junction 81) : {LgrstOpn;}
  (junction 73) -> (junction 87)
  (junction 81) -> (junction 73)
  data: IfVeSMSuSecRwLtStBkReclnUpwdDnwdPos input; IfVeSMSuSecRwLtStLgrstOtwdInwdPos input; IfVeSMSuSecRwLtStLgrstUpwdDnwdPos input; SecRwLtStBkReclnStgDone input; SecRwLtStFrwdBkwdStgDone input; SecRwLtStLgrstOtwdInwdStgDone input; SecRwLtStLgrstUpwdDnwdStgDone input; ThdRwLtStBkReclnStgDone input; ThdRwLtStFwdBkwdStgDone input; VIPLR2LBkReclnUpwdDnwdTrgtPos input; VIPLR2LFwdBkwdTrgtPos input; VIPLR2LLgrstInwdOtwdTrgtPos input; VIPLR2LLgrstUpwdDnwdTrgtPos input; SecRwLtStBkReclnEn output boolean; SecRwLtStFrwdBkwdEn output boolean; SecRwLtStLgrstOtwdInwdEn output boolean; ThdRwLtStBkReclnEn output boolean; ThdRwLtStFwdBkwdEn output boolean; SecRwLtStLgrstUpwdDnwdEn output boolean
  events: LgrstOpn output FUNCTION_CALL_EVENT
